simulink model "GridConnected"  (R2022b)
settings: Solver=ode23tb  StartTime=0.0  StopTime=24*3600*365*3  FixedStep=60  RelTol=1e-3
values from neighbouring files (symbols this model uses):
  Fnom = 50    [run_test.m]
  Tsample = 60    [run_test.m]
  Vnom = sqrt(3)*230    [run_test.m]
libraries: ET3036TU_model_library_2021b x6, simulink x6, spsThreePhaseDynamicLoadLib x2, spspowerguiLib x1
settings Model: Creator=nkpanda  LastModifiedBy=jeroen
settings SolverCC: ZeroCrossAlgorithm=Adaptive
settings DebuggingCC: IgnoredZcDiagnostic=none  UnconnectedInputMsg=warning  UnconnectedOutputMsg=warning  UnconnectedLineMsg=warning
settings ModelReferenceCC: EnableRefExpFcnMdlSchedulingChecks=on
settings RTWCC: DLArmComputeVersion=19.05

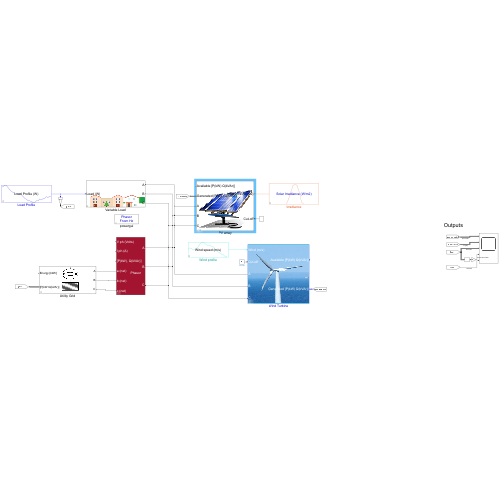
[thumbnail: Simulink's stored preview of the top-level diagram]
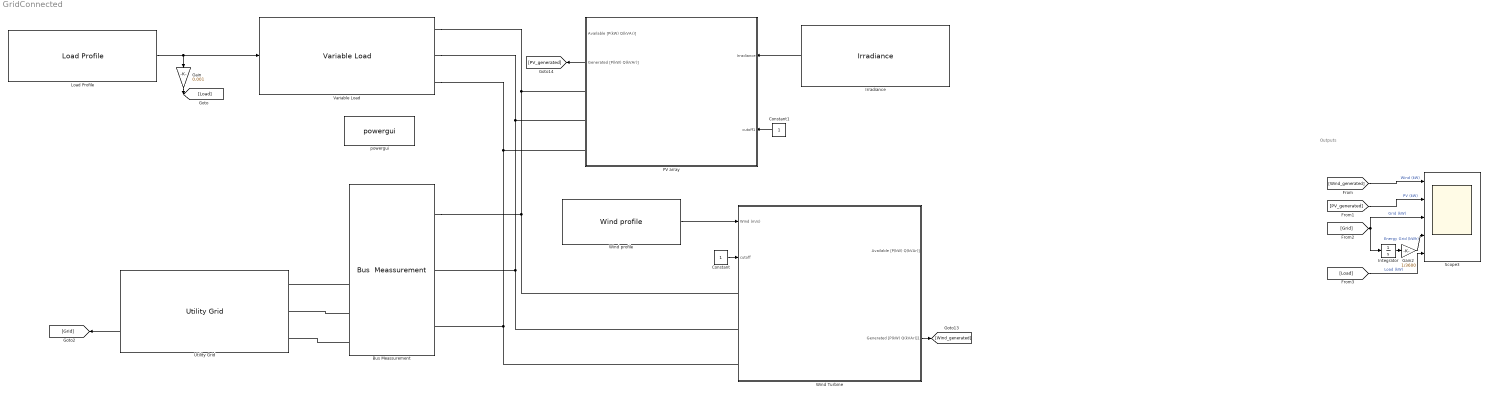
== system GridConnected ==
  note: Outputs
  "Bus Meassurement " : ET3036TU_model_library_2021b/Bus  Meassurement 
  Constant : Constant
  Constant1 : Constant
  Gain : Gain  Gain=0.001
  Gain2 : Gain  Gain=1/3600
  Integrator : Integrator
  Irradiance : ET3036TU_model_library_2021b/Irradiance
  Load Profile : ET3036TU_model_library_2021b/Load Profile
  "PV array " : Subsystem  AncestorBlock=ET3036TU_model_library_2021b/PV array  mask(PV farm){Efficiency=0.2, Area=522.71, Vnom=Vnom, fnom=Fnom}
      mask prompts: Efficiency "Total efficiency (fraction)"; Area "Area (m2)"; Vnom "Rated Line voltage (Vrms)"; fnom "Rated frequency (Hz):"
      mask help: The product of the efficiency, the area covered by the PV farm and the irradiance in W/m2 will give you the power generated by the PV farm.
      settings: LibrarySourceBlock=ET3036TU_model_library_2021b/PV array
      mask Display:
      | color('white')
      | image(imread('pv.jpg'))
      | 
      | color('black')
      | port_label('RConn',1,'A')
      | port_label('RConn',2,'B')
      | port_label('RConn',3,'C')
      | port_label('output',1,'Available [P(kW) Q(kVAr)]')
      | port_label('output',2,'Generated [P(kW) Q(kVAr)]')
      | 
      | port_label('input',1,'Irradiance (W/m2)')
      | port_label('input',2,'Cut-off')
  Scope3 : Scope  NumInputPorts=5
  Utility Grid : ET3036TU_model_library_2021b/Utility Grid
  Variable Load : ET3036TU_model_library_2021b/Variable Load  PF=1  Load0=0
  "Wind Turbine " : Subsystem  AncestorBlock=ET3036TU_model_library_2021b/Wind Turbine  mask{Unom=15, Umax=25, Umin=3, Pselect=1: Simple Cubic Power, fnom=Fnom, Vnom=Vnom, Pnom=110, rp=5, Cp=16/27, rho=1.225, Uvec=1:1:30, Pvec=[0,0,0,0,21359.3750000000,58193.5000000000,104316.125000000,157104.500000000,213935.875000000,272187.500000000,329236.625000000,382460.500000000,429236.375000000,466941.500000000,492953.125000000,500000,500000,500000,500000,500000,500000,500000,500000,500000,500000,0,0,0,0,0], Tp=1, Tq=0.1, ReactP=0}
      mask prompts: Unom "Nominal Wind Speed [m/s]"; Umax "Maximum Operating Wind [m/s]"; Umin "Minimum Operating Wind [m/s]"; Pselect "Wind Turbine Power Model"; fnom "Nominal frequency (Hz):"; Vnom "Nominal phae-to-phase voltage (Vrms)"; Pnom "Nominal Power, [kW]"; rp "Blade Radius, r [m]"; Cp "Performance Coefficient, Cp"; rho "Air Density, rho [kg/m^3]"; Uvec "Wind Vec [m/s]"; Pvec "Power Vec [W]"; Tp "Active Power Dynamics, Tp [s]"; Tq "Reactive Power Dynamics, Tq [s]"; ReactP "Reactive Power Percentage [%]"
      mask help:
      | Simple Wind Turbine that serves as an Active and Reactive Power Source depending on the Wind Power Curve.
      |
      | The Wind Turbine Power Curve can be defined by one of three models:
      | 1: Simple cubic power curve
      | 2: Physical wind turbine parameters
      | 3: Look-up table (from a wind turbine data sheet).
      |
      | Cutoff takes value 1 or 0. 1 denotes manual forced cut-off od wind power generation even though potnetial wind power is available
      | The 'General' and 'Dynamics' tabs apply to all models.
      mask init:
      | A = pi*rp^2;
      | 
      | if Pselect == 1,
      |     Pmax = Pnom*1e3;
      | elseif Pselect == 2,
      |     Pmax = 1/2*rho*Cp*A*Umax^3;
      | else
      |     Pmax = max(Pvec);
      | end
      | Qmax = (ReactP/100)*Pmax;
      settings: LibrarySourceBlock=ET3036TU_model_library_2021b/Wind Turbine
      mask TypeOptions Pselect: 1: Simple Cubic Power | 2: Physical parameters | 3: Look-up Fit
      mask DialogControl Container4 Prompt: General
      mask DialogControl Container16 Prompt: Turbine
      mask DialogControl Container10 Prompt: Electrical
      mask DialogControl Container12 Prompt: 1: Cubic
      mask DialogControl Container9 Prompt: 2: Physical
      mask DialogControl Container7 Prompt: 3: Lookup
      mask DialogControl Container8 Prompt: Dynamics
      mask Display:
      | image(imread('eolienne.bmp'))
      | 
      | color('white')
      | port_label('LConn',1,'A')
      | port_label('LConn',2,'B')
      | port_label('LConn',3,'C')
      | 
      | port_label('output',1,'Available [P(kW) Q(kVAr)]')
      | port_label('output',2,'Generated [P(kW) Q(kVAr)]')
      | port_label('input',1,'Wind (m/s)')
      | port_label('input',2,'Cut-off')
  Wind profile : ET3036TU_model_library_2021b/Wind profile
  powergui : spspowerguiLib/powergui  Priority=1  SimulationMode=Phasor  SampleTime=Tsample  frequency=Fnom  Iterations=50  frequencyindice=50  Pbase=100e6  ErrMax=1e-4  UnitsV=kV  UnitsW=MW  buscounter=0  FunctionMessages=off  echomessages=off  EnableUseOfTLC=off  CurrentSourceSwitches=off  DisableSnubberDevices=off  DisableRonSwitches=off  DisableVfSwitches=off  DisplayEquations=off  AutomaticDiscreteSolvers=off  SolverType=Tustin/Backward Euler (TBE)  Interpol=off  ExternalGateDelay=off  methode=off  Ts=100  x0status=blocks  SPID=on  SwTol=0  HookPort=off  NonlinearTolerance=1e-4  nMaxIteration=100  ContinueOnMaxIteration=off  RestoreLinks=warning  ResistiveCurrentMeasurement=off  Frange=[0:2:500]  Ylog=off  Xlog=on  ShowGrid=off  save=off  variable=ZData  structure=0  ZoomFFT=off  StartTime=0.0  cycles=1  DisplayStyle=1  fundamental=60  FreqAxis=off  MaxFrequency=1000  frequencyindicesteady=1  RmsSteady=1  display=off
  wires:
  Load Profile/1 -> Gain/1, Variable Load/1
  Irradiance/1 -> "PV array "/1(Irradiance)
  Gain/1 -> [Load]
  Constant/1 -> "Wind Turbine "/2(cutoff)
  "Wind Turbine "/2(Generated [P(kW) Q(kVAr)]1) -> [Wind_generated]
  "PV array "/2(Generated [P(kW) Q(kVAr)]) -> [PV_generated]
  Wind profile/1 -> "Wind Turbine "/1(Wind (m/s))
  Utility Grid/2 -> [Grid]
  Constant1/1 -> "PV array "/2(cutoff1)
  [Wind_generated] -> Scope3/1  "Wind (kW)"
  [PV_generated] -> Scope3/2  "PV (kW)"
  [Grid] -> Integrator/1, Scope3/3  "Grid (kW)"
  Gain2/1 -> Scope3/4  "Energy Grid (kWh)"
  Integrator/1 -> Gain2/1
  [Load] -> Scope3/5  "Load (kW)"
  connections:
  "Bus Meassurement "/RConn1 -- Utility Grid/LConn1
  "Bus Meassurement "/RConn2 -- Utility Grid/LConn2
  "Bus Meassurement "/RConn3 -- Utility Grid/LConn3
  "PV array "/RConn2 -- "Wind Turbine "/LConn2 -- "Bus Meassurement "/LConn2 -- Variable Load/RConn2
  "Bus Meassurement "/LConn1 -- "Wind Turbine "/LConn1 -- Variable Load/RConn1 -- "PV array "/RConn1
  "PV array "/RConn3 -- "Wind Turbine "/LConn3 -- "Bus Meassurement "/LConn3 -- Variable Load/RConn3

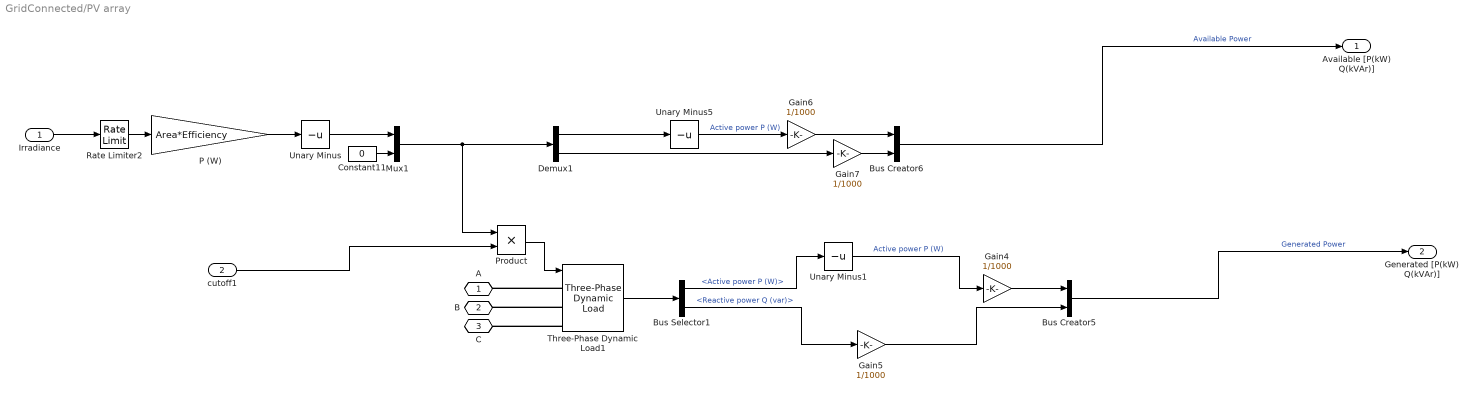
== system GridConnected/PV array  ==
  Irradiance : Inport
  cutoff1 : Inport  Port=2
  Bus Creator5 : BusCreator  Inputs=2
  Bus Creator6 : BusCreator  Inputs=2
  Bus Selector1 : BusSelector  OutputSignals=Active power P (W),Reactive power Q (var)
  Constant11 : Constant  Value=0
  Demux1 : Demux  Outputs=2
  Gain{4..7} (4 alike) : Gain  Gain=1/1000
  Mux1 : Mux  Inputs=2
  P (W) : Gain  Gain=Area*Efficiency
  Product : Product
  Rate Limiter2 : RateLimiter  RisingSlewLimit=1e4  FallingSlewLimit=-1e4  SampleTimeMode=inherited
  Three-Phase Dynamic Load1 : spsThreePhaseDynamicLoadLib/Three-Phase Dynamic Load  NominalVoltage=[Vnom fnom]  ActiveReactivePowers="[ 0  0]"  PositiveSequence=[Vnom 0]  ExternalControl=on  NpNq=[1.3 2]  TimeConstants="[0  0  0  0]"  MinimumVoltage=0.7  Tfilter=1e-4  LoadFlowParameters=[4,0,0,0,0]
  Unary Minus : UnaryMinus
  Unary Minus1 : UnaryMinus
  Unary Minus5 : UnaryMinus
  A : PMIOPort  Side=Right
  B : PMIOPort  Port=2  Side=Right
  C : PMIOPort  Port=3  Side=Right
  Available [P(kW) Q(kVAr)] : Outport  VectorParamsAs1DForOutWhenUnconnected=off
  Generated [P(kW) Q(kVAr)] : Outport  Port=2  VectorParamsAs1DForOutWhenUnconnected=off
  wires:
  Bus Creator5/1 -> Generated [P(kW) Q(kVAr)]/1  "Generated Power"
  Rate Limiter2/1 -> P (W)/1
  Constant11/1 -> Mux1/2
  Unary Minus/1 -> Mux1/1
  P (W)/1 -> Unary Minus/1
  Irradiance/1 -> Rate Limiter2/1
  Bus Selector1/1 -> Unary Minus1/1  "<Active power P (W)>"
  Unary Minus1/1 -> Gain4/1  "Active power P (W)"
  Three-Phase Dynamic Load1/1 -> Bus Selector1/1
  Bus Selector1/2 -> Gain5/1  "<Reactive power Q (var)>"
  Gain4/1 -> Bus Creator5/1
  Gain5/1 -> Bus Creator5/2
  Demux1/1 -> Unary Minus5/1
  Gain6/1 -> Bus Creator6/1
  Demux1/2 -> Gain7/1
  Unary Minus5/1 -> Gain6/1  "Active power P (W)"
  Gain7/1 -> Bus Creator6/2
  Bus Creator6/1 -> Available [P(kW) Q(kVAr)]/1  "Available Power"
  Product/1 -> Three-Phase Dynamic Load1/1
  Mux1/1 -> Product/1, Demux1/1
  cutoff1/1 -> Product/2
  connections:
  Three-Phase Dynamic Load1/LConn2 -- B/RConn1
  Three-Phase Dynamic Load1/LConn1 -- A/RConn1
  Three-Phase Dynamic Load1/LConn3 -- C/RConn1

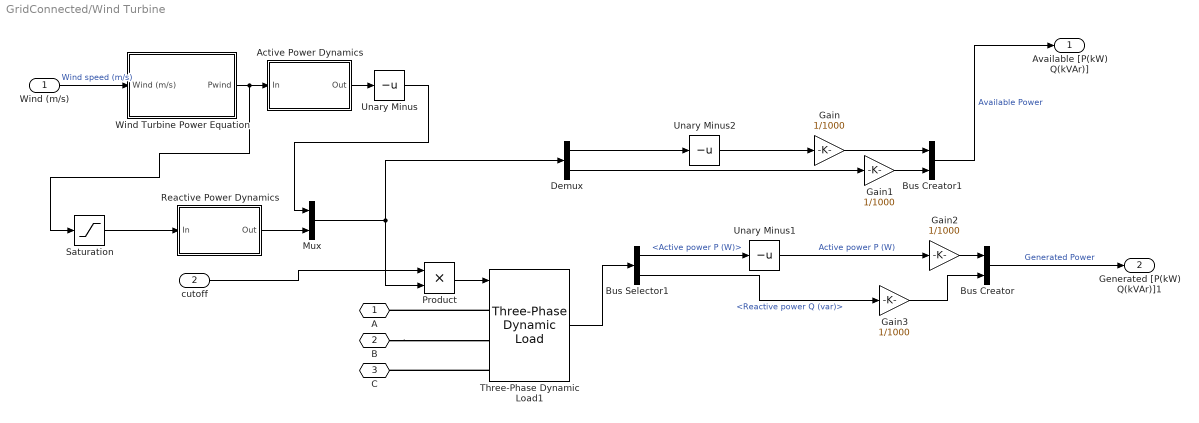
== system GridConnected/Wind Turbine  ==
  Wind (m/s) : Inport
  cutoff : Inport  Port=2
  Active Power Dynamics : Subsystem  VariantControl=T6NotZero
      mask Display: disp('1 / (1 + s T_P)','texmode','on');
  Bus Creator : BusCreator  Inputs=2
  Bus Creator1 : BusCreator  Inputs=2
  Bus Selector1 : BusSelector  OutputSignals=Active power P (W),Reactive power Q (var)
  Demux : Demux  Outputs=2
  Gain{,1..3} (4 alike) : Gain  Gain=1/1000
  Mux : Mux  Inputs=2
  Product : Product
  Reactive Power Dynamics : Subsystem  VariantControl=T6NotZero
      mask Display: disp('1 / (1 + s T_Q)','texmode','on');
  Saturation : Saturate  UpperLimit=Qmax  LowerLimit=-Qmax
  Three-Phase Dynamic Load1 : spsThreePhaseDynamicLoadLib/Three-Phase Dynamic Load  NominalVoltage=[Vnom fnom]  ActiveReactivePowers="[ 0  0]"  PositiveSequence=[Vnom 0]  ExternalControl=on  NpNq=[1.3 2]  TimeConstants="[0  0  0  0]"  MinimumVoltage=0.7  Tfilter=1e-4  LoadFlowParameters=[4,0,0,0,0]
  Unary Minus : UnaryMinus
  Unary Minus1 : UnaryMinus
  Unary Minus2 : UnaryMinus
  Wind Turbine Power Equation : Subsystem
  A : PMIOPort  Side=Left
  B : PMIOPort  Port=2  Side=Left
  C : PMIOPort  Port=3  Side=Left
  Available [P(kW) Q(kVAr)] : Outport  VectorParamsAs1DForOutWhenUnconnected=off
  Generated [P(kW) Q(kVAr)]1 : Outport  Port=2  VectorParamsAs1DForOutWhenUnconnected=off
  wires:
  Bus Selector1/2 -> Gain3/1  "<Reactive power Q (var)>"
  Unary Minus1/1 -> Gain2/1  "Active power P (W)"
  Bus Selector1/1 -> Unary Minus1/1  "<Active power P (W)>"
  Three-Phase Dynamic Load1/1 -> Bus Selector1/1
  Unary Minus/1 -> Mux/1
  Active Power Dynamics/1(Out) -> Unary Minus/1
  Wind Turbine Power Equation/1(Pwind) -> Saturation/1, Active Power Dynamics/1(In)
  Reactive Power Dynamics/1(Out) -> Mux/2
  Saturation/1 -> Reactive Power Dynamics/1(In)
  Wind (m/s)/1 -> Wind Turbine Power Equation/1(Wind (m/s))  "Wind speed (m/s)"
  Mux/1 -> Demux/1, Product/2
  Product/1 -> Three-Phase Dynamic Load1/1
  cutoff/1 -> Product/1
  Demux/1 -> Unary Minus2/1
  Demux/2 -> Gain1/1
  Unary Minus2/1 -> Gain/1
  Gain/1 -> Bus Creator1/1
  Gain1/1 -> Bus Creator1/2
  Gain2/1 -> Bus Creator/1
  Gain3/1 -> Bus Creator/2
  Bus Creator1/1 -> Available [P(kW) Q(kVAr)]/1  "Available Power"
  Bus Creator/1 -> Generated [P(kW) Q(kVAr)]1/1  "Generated Power"
  connections:
  B/RConn1 -- Three-Phase Dynamic Load1/LConn2
  Three-Phase Dynamic Load1/LConn3 -- C/RConn1
  Three-Phase Dynamic Load1/LConn1 -- A/RConn1

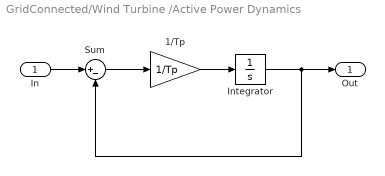
== system GridConnected/Wind Turbine /Active Power Dynamics ==
  In : Inport
  1/Tp : Gain  Gain=1/Tp
  Integrator : Integrator
  Sum : Sum  Inputs=|+-
  Out : Outport  VectorParamsAs1DForOutWhenUnconnected=off
  wires:
  Integrator/1 -> Out/1, Sum/2
  In/1 -> Sum/1
  1/Tp/1 -> Integrator/1
  Sum/1 -> 1/Tp/1

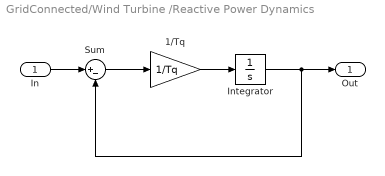
== system GridConnected/Wind Turbine /Reactive Power Dynamics ==
  In : Inport
  1/Tq : Gain  Gain=1/Tq
  Integrator : Integrator
  Sum : Sum  Inputs=|+-
  Out : Outport  VectorParamsAs1DForOutWhenUnconnected=off
  wires:
  Sum/1 -> 1/Tq/1
  1/Tq/1 -> Integrator/1
  In/1 -> Sum/1
  Integrator/1 -> Sum/2, Out/1

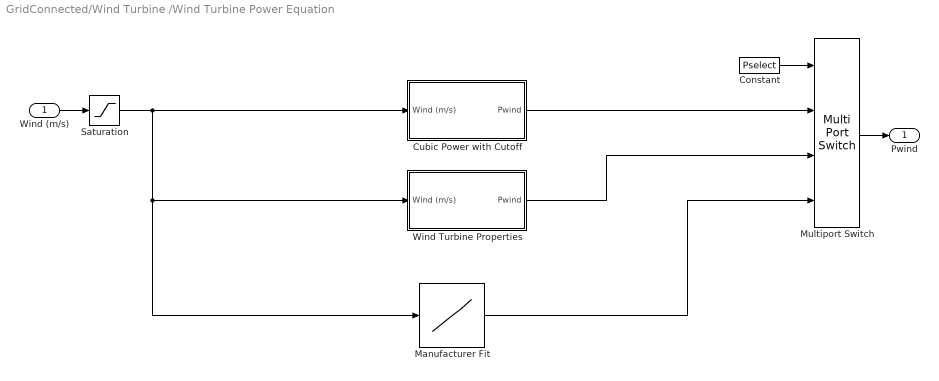
== system GridConnected/Wind Turbine /Wind Turbine Power Equation ==
  Wind (m/s) : Inport
  Constant : Constant  Value=Pselect
  Cubic Power with Cutoff : Subsystem
  Manufacturer Fit : Lookup_n-D  NumberOfTableDimensions=1  BreakpointsForDimension1=Uvec  Table=Pvec  ExtrapMethod=Clip  InternalRulePriority=Speed  RndMeth=Simplest
  Multiport Switch : MultiPortSwitch  SaturateOnIntegerOverflow=off  InputSameDT=off
  Saturation : Saturate  UpperLimit=inf  LowerLimit=0  ZeroCross=off
      settings: AttributesFormatString=|
      | %<UpperLimit>
      | %<LowerLimit>
  Wind Turbine Properties : Subsystem
  Pwind : Outport  VectorParamsAs1DForOutWhenUnconnected=off
  wires:
  Manufacturer Fit/1 -> Multiport Switch/4
  Saturation/1 -> Manufacturer Fit/1, Wind Turbine Properties/1(Wind (m/s)), Cubic Power with Cutoff/1(Wind (m/s))
  Constant/1 -> Multiport Switch/1
  Multiport Switch/1 -> Pwind/1
  Wind (m/s)/1 -> Saturation/1
  Wind Turbine Properties/1(Pwind) -> Multiport Switch/3
  Cubic Power with Cutoff/1(Pwind) -> Multiport Switch/2

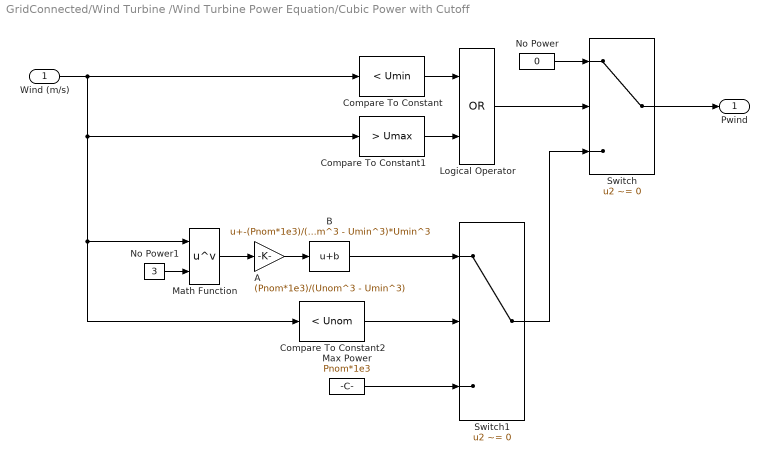
== system GridConnected/Wind Turbine /Wind Turbine Power Equation/Cubic Power with Cutoff ==
  Wind (m/s) : Inport
  A : Gain  Gain=(Pnom*1e3)/(Unom^3 - Umin^3)
  B : Bias  Bias=-(Pnom*1e3)/(Unom^3 - Umin^3)*Umin^3  SaturateOnIntegerOverflow=off
  Compare To Constant : simulink/Logic and Bit Operations/Compare To Constant  relop=<  const=Umin  OutDataTypeStr=boolean
  Compare To Constant1 : simulink/Logic and Bit Operations/Compare To Constant  relop=>  const=Umax  OutDataTypeStr=boolean
  Compare To Constant2 : simulink/Logic and Bit Operations/Compare To Constant  relop=<  const=Unom  OutDataTypeStr=boolean
  Logical Operator : Logic  Operator=OR  AllPortsSameDT=off  OutDataTypeStr=boolean
  Math Function : Math  Operator=pow  SignedPower=on
  Max Power : Constant  Value=Pnom*1e3
  No Power : Constant  Value=0
  No Power1 : Constant  Value=3
  Switch : Switch  Criteria=u2 ~= 0  ZeroCross=off  SaturateOnIntegerOverflow=off  InputSameDT=off
  Switch1 : Switch  Criteria=u2 ~= 0  ZeroCross=off  SaturateOnIntegerOverflow=off  InputSameDT=off
  Pwind : Outport  VectorParamsAs1DForOutWhenUnconnected=off
  wires:
  Compare To Constant/1 -> Logical Operator/1
  Switch/1 -> Pwind/1
  Logical Operator/1 -> Switch/2
  A/1 -> B/1
  Wind (m/s)/1 -> Compare To Constant2/1, Math Function/1, Compare To Constant1/1, Compare To Constant/1
  Max Power/1 -> Switch1/3
  Switch1/1 -> Switch/3
  No Power/1 -> Switch/1
  No Power1/1 -> Math Function/2
  Math Function/1 -> A/1
  Compare To Constant1/1 -> Logical Operator/2
  Compare To Constant2/1 -> Switch1/2
  B/1 -> Switch1/1

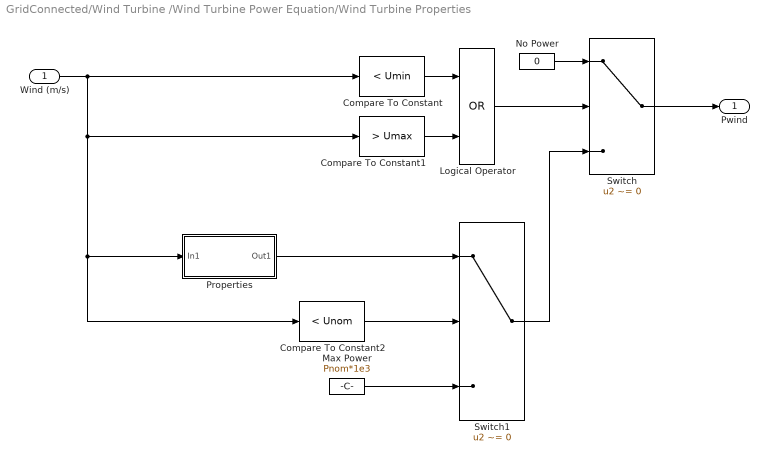
== system GridConnected/Wind Turbine /Wind Turbine Power Equation/Wind Turbine Properties ==
  Wind (m/s) : Inport
  Compare To Constant : simulink/Logic and Bit Operations/Compare To Constant  relop=<  const=Umin  OutDataTypeStr=boolean
  Compare To Constant1 : simulink/Logic and Bit Operations/Compare To Constant  relop=>  const=Umax  OutDataTypeStr=boolean
  Compare To Constant2 : simulink/Logic and Bit Operations/Compare To Constant  relop=<  const=Unom  OutDataTypeStr=boolean
  Logical Operator : Logic  Operator=OR  AllPortsSameDT=off  OutDataTypeStr=boolean
  Max Power : Constant  Value=Pnom*1e3
  No Power : Constant  Value=0
  Properties : Subsystem
  Switch : Switch  Criteria=u2 ~= 0  ZeroCross=off  SaturateOnIntegerOverflow=off  InputSameDT=off
  Switch1 : Switch  Criteria=u2 ~= 0  ZeroCross=off  SaturateOnIntegerOverflow=off  InputSameDT=off
  Pwind : Outport  VectorParamsAs1DForOutWhenUnconnected=off
  wires:
  Properties/1(Out1) -> Switch1/1
  Compare To Constant2/1 -> Switch1/2
  Compare To Constant1/1 -> Logical Operator/2
  No Power/1 -> Switch/1
  Switch1/1 -> Switch/3
  Max Power/1 -> Switch1/3
  Wind (m/s)/1 -> Compare To Constant/1, Compare To Constant1/1, Properties/1(In1), Compare To Constant2/1
  Logical Operator/1 -> Switch/2
  Switch/1 -> Pwind/1
  Compare To Constant/1 -> Logical Operator/1

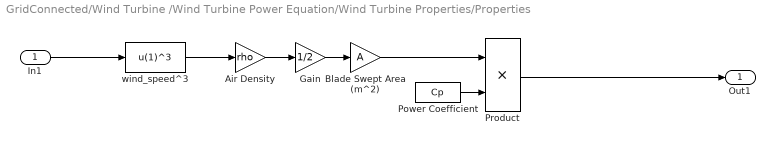
== system GridConnected/Wind Turbine /Wind Turbine Power Equation/Wind Turbine Properties/Properties ==
  In1 : Inport
  Air Density : Gain  Gain=rho
  Blade Swept Area (m^2) : Gain  Gain=A
  Gain : Gain  Gain=1/2
  Power Coefficient : Constant  Value=Cp
  "Product " : Product  SaturateOnIntegerOverflow=on  OutDataTypeStr=Inherit: Same as first input
  wind_speed^3 : Fcn  Expr=u(1)^3
  Out1 : Outport  VectorParamsAs1DForOutWhenUnconnected=off
  wires:
  Blade Swept Area (m^2)/1 -> "Product "/1
  wind_speed^3/1 -> Air Density/1
  Power Coefficient/1 -> "Product "/2
  In1/1 -> wind_speed^3/1
  Air Density/1 -> Gain/1
  "Product "/1 -> Out1/1
  Gain/1 -> Blade Swept Area (m^2)/1
